simulink model "ECE141Q3"  (R2021b)
settings: Solver=VariableStepAuto  StartTime=0.0  StopTime=10.0  RelTol=1e-3
settings Model: Creator=ineshchakrabarti  LastModifiedBy=ineshchakrabarti
settings DataIOCC: Refine=100

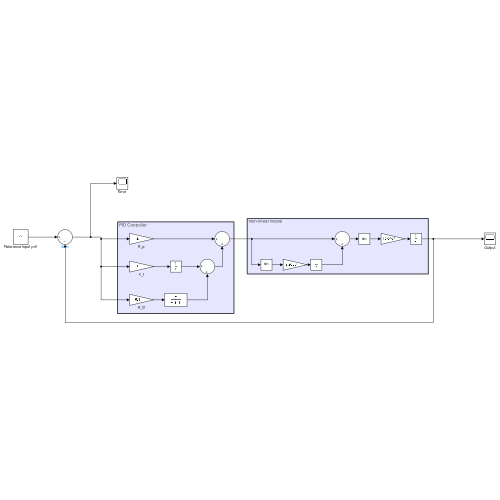
[thumbnail: Simulink's stored preview of the top-level diagram]
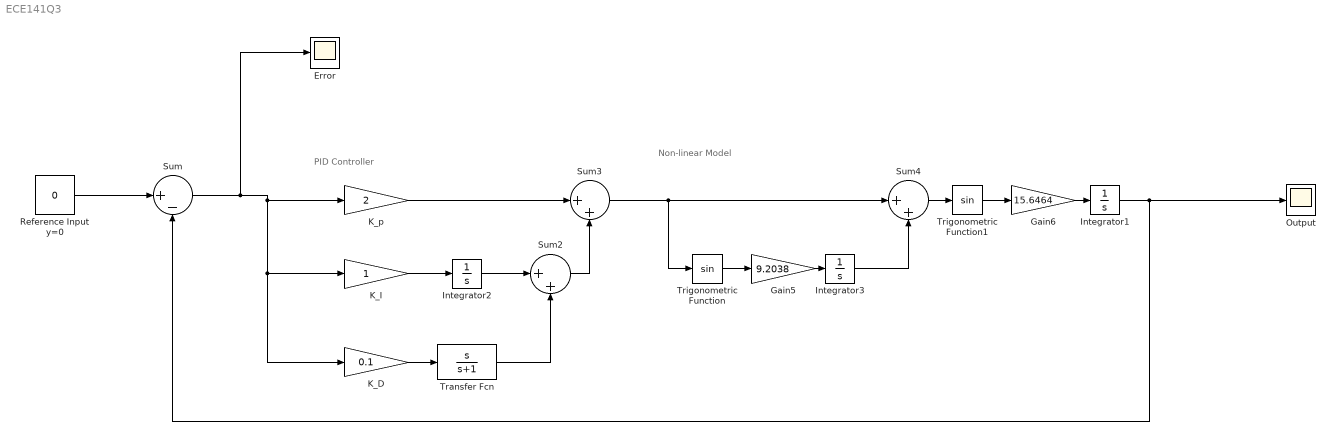
== system ECE141Q3 ==
  note: Non-linear Model
  note: PID Controller
  Error : Scope
  Gain5 : Gain  Gain=9.2038
  Gain6 : Gain  Gain=15.6464
  Integrator1 : Integrator  InitialCondition=0.6
  Integrator2 : Integrator
  Integrator3 : Integrator  InitialCondition=0.8
  K_D : Gain  Gain=0.1
  K_I : Gain
  K_p : Gain  Gain=2
  Output : Scope
  Reference Input y=0 : Constant  Value=0
  Sum : Sum  Inputs=|+-
  Sum2 : Sum  Inputs=|++
  Sum3 : Sum  Inputs=|++
  Sum4 : Sum  Inputs=|++
  Transfer Fcn : TransferFcn  Numerator=[1 0]  Denominator=[1 1]
  Trigonometric Function : Trigonometry
  Trigonometric Function1 : Trigonometry
  wires:
  Transfer Fcn/1 -> Sum2/2
  Sum2/1 -> Sum3/2
  K_I/1 -> Integrator2/1
  Sum/1 -> Error/1, K_I/1, K_D/1, K_p/1
  Integrator2/1 -> Sum2/1
  K_p/1 -> Sum3/1
  K_D/1 -> Transfer Fcn/1
  Sum3/1 -> Sum4/1, Trigonometric Function/1
  Gain5/1 -> Integrator3/1
  Gain6/1 -> Integrator1/1
  Integrator1/1 -> Output/1, Sum/2
  Reference Input y=0/1 -> Sum/1
  Trigonometric Function/1 -> Gain5/1
  Sum4/1 -> Trigonometric Function1/1
  Trigonometric Function1/1 -> Gain6/1
  Integrator3/1 -> Sum4/2
